simulink model "TrayectoriaObstaculos"  (R2023b)
settings: Solver=FixedStepAuto  StartTime=0.0  StopTime=150  RelTol=1e-3
model workspace (MAT data in the model file):
  d = 0.2
libraries: robotalgslib x1
settings Model: ExtModeTrigDuration=2  Creator=ricfe  LastModifiedBy=ricfe
settings OptimizationCC: EnhancedBackFolding=on  PassReuseOutputArgsAs=Individual arguments  ZeroExternalMemoryAtStartup=off  ZeroInternalMemoryAtStartup=off  MaxStackSize=64  OptimizeBlockOrder=speed  DifferentSizesBufferReuse=on  EfficientTunableParamExpr=on
settings DebuggingCC: ParameterTunabilityLossMsg=error
settings HardwareCC: ProdBitPerInt=16  ProdBitPerPointer=16  ProdBitPerSizeT=16  ProdBitPerPtrDiffT=16  ProdLargestAtomicFloat=None  ProdWordSize=8  ProdHWDeviceType=Atmel->AVR  UseEmbeddedCoderFeatures=off
settings SFSimCC: MATLABDynamicMemAlloc=off
settings RTWCC: Description=Embedded Coder  SystemTargetFile=ert.tlc  HardwareBoard=Arduino Mega 2560  TemplateMakefile=ert_default_tmf  Toolchain=Arduino AVR
settings CodeAppCC: ForceParamTrailComments=on  IgnoreCustomStorageClasses=off  OperatorAnnotations=on  SimulinkDataObjDesc=on  SFDataObjDesc=on  InsertBlockDesc=on
settings ERTTargetCC: SupportContinuousTime=on  SupportNonInlinedSFcns=on  SupportVariableSizeSignals=on  ExtModeTransport=3  ExtModeStaticAlloc=on  ExtModeAutomaticAllocSize=off  ExtModeStaticAllocSize=2048  ExtModeMexFile=ext_xcp  ExtModeIntrfLevel=Level2 - Open

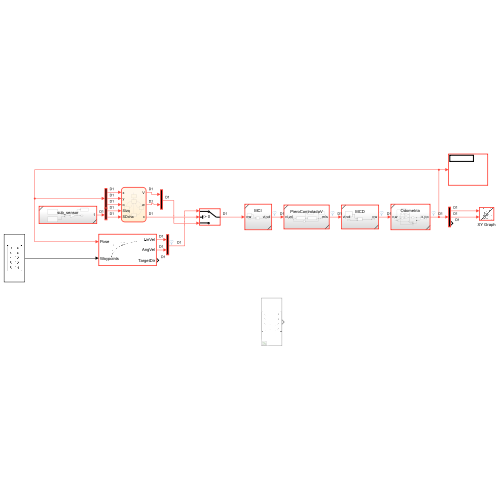
[thumbnail: Simulink's stored preview of the top-level diagram]
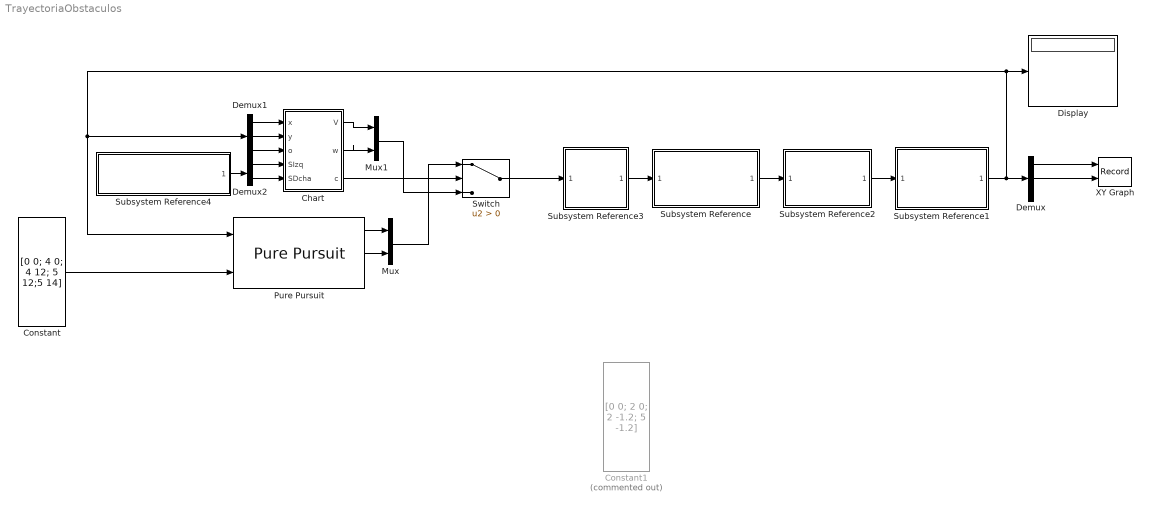
== system TrayectoriaObstaculos ==
  Chart : Stateflow chart  TreatAsAtomicUnit=on
  Constant : Constant  Value=[0 0; 4 0; 4 12; 5 12;5 14]
  Constant1 : Constant  Commented=on  Value=[0 0; 2 0; 2 -1.2; 5 -1.2]
  Demux : Demux  Outputs=3
  Demux1 : Demux  Outputs=3
  Demux2 : Demux  Outputs=2
  Display : Display
  Mux : Mux  Inputs=2
  Mux1 : Mux  Inputs=2
  Pure Pursuit : robotalgslib/Pure Pursuit  DesiredLinearVelocity=0.205  MaxAngularVelocity=0.75  LookaheadDistance=0.15  TargetDirPort=on  SimulateUsing=Code generation
      settings: LibrarySourceBlock=navlib/Control Algorithms/Pure Pursuit
  Subsystem Reference : Subsystem  ReferencedSubsystem=PieroControladoV
  Subsystem Reference1 : Subsystem  ReferencedSubsystem=Odometria
  Subsystem Reference2 : Subsystem  ReferencedSubsystem=MCD
  Subsystem Reference3 : Subsystem  ReferencedSubsystem=MCI
  Subsystem Reference4 : Subsystem  ReferencedSubsystem=sub_sensor
  Switch : Switch  Criteria=u2 > Threshold  SaturateOnIntegerOverflow=off  InputSameDT=off
  XY Graph : Record  FileSettingsInternal="{\"entries\":[{\"content\":{\"excelSettings\":{\"content\":{},\"type\":\"Streamout.ExcelSettings\"}},\"type\":\"Streamout.FileSettingStorage\",\"uuid\":\"\"}],\"packageUris\":[\"http:\\/\\/schema.mathworks.com\\/mf0\\/streamout_blocks\\/R2020a\"],\"version\":\"1.0\"}"  Layout=[1 1]  SignalsInternal="{\"entries\":[{\"content\":{\"signals\":[{\"content\":{\"blockPath\":[],\"dimensions\":[1],\"domain\":\"\",\"lineColor\":\"#0072bd\",\"plots\":[ 1 ],\"port\":1,\"sid\":[\"\"],\"signalID\":1,\"signalName\":\"Demux:1\"},\"type\":\"RecordBlkView.Signal\",\"uuid\":\"\"},{\"content\":{\"blockPath\":[],\"dimensions\":[1],\"domain\":\"\",\"lineColor\":\"#d95319\",\"plots\":[ 1 ],\"port\":2,\"sid\":[\"\"],\"signalID\":2,\"signalName\":\"Demux:2\"},\"type\":\"RecordBlkView.Signal\",\"uuid\":\"\"}]},\"type\":\"RecordBlkView.InputSignals\",\"uuid\":\"\"}],\"packageUris\":[\"http:\\/\\/schema.mathworks.com\\/mf0\\/streamout_blocks\\/R2020a\"],\"version\":\"1.0\"}"  VisualizationBindings="{\"xyplotplugin\":{\"info\":[{\"series\":[{\"bindingParametersList\":[{\"parameter\":\"X-Axis\",\"signalID\":1,\"signalName\":\"Demux:1\"},{\"parameter\":\"Y-Axis\",\"signalID\":2,\"signalName\":\"Demux:2\"}],\"seriesID\":0},{\"bindingParametersList\":[{\"parameter\":\"X-Axis\",\"signalID\":2,\"signalName\":\"Demux:2\"}],\"seriesID\":1}],\"subplotID\":1}]}}"  CompatibilityTag=XY
  wires:
  Constant/1 -> Pure Pursuit/2
  Subsystem Reference2/1 -> Subsystem Reference1/1
  Pure Pursuit/2 -> Mux/2
  Pure Pursuit/1 -> Mux/1
  Subsystem Reference/1 -> Subsystem Reference2/1
  Demux/1 -> XY Graph/1
  Subsystem Reference3/1 -> Subsystem Reference/1
  Demux/2 -> XY Graph/2
  Subsystem Reference1/1 -> Display/1, Demux1/1, Pure Pursuit/1, Demux/1
  Demux1/1 -> Chart/1(x)
  Chart/1(V) -> Mux1/1
  Demux1/3 -> Chart/3(o)
  Demux1/2 -> Chart/2(y)
  Chart/3(c) -> Switch/2
  Chart/2(w) -> Mux1/2
  Demux2/1 -> Chart/4(SIzq)
  Demux2/2 -> Chart/5(SDcha)
  Subsystem Reference4/1 -> Demux2/1
  Switch/1 -> Subsystem Reference3/1
  Mux/1 -> Switch/1
  Mux1/1 -> Switch/3

== stateflow chart TrayectoriaObstaculos/Chart ==
  state Inicio
    entry:
    V = 0;
    w = 0;
    c = 0;
  state SinObstaculos
    entry:
    V = 0;
    w = 0;
    c = 1;
  state ObstaculoIzq
    entry:
    V = 0.1;
    w = -pi/4;
    c = 0;
  state ObstaculoDcha
    entry:
    V = 0.1;
    w = pi/4;
    c = 0;
  state ObstaculoFrente
    entry:
    V = 0;
    w = pi/2;
    c = 0;
  (default) -> Inicio
  Inicio -> SinObstaculos
  SinObstaculos -> ObstaculoDcha [order 1] : [SDcha < 20]
  SinObstaculos -> ObstaculoIzq [order 2] : [SIzq < 20]
  ObstaculoIzq -> SinObstaculos [order 2] : after(1,sec)
  ObstaculoFrente -> SinObstaculos : after(1.5,sec)
  ObstaculoDcha -> SinObstaculos [order 2] : after(1,sec)
  ObstaculoIzq -> ObstaculoFrente [order 1] : [SDcha < 20]
  ObstaculoDcha -> ObstaculoFrente [order 1] : [SIzq < 20]
  data: x input; y input; V output double size=1; w output double size=1; o input; c output double size=1; SIzq input; SDcha input
